simulink model "mrand_bpsk_1u_mp"  (Simulink 6.0)
settings: Solver=ode45  StartTime=0.0  StopTime=" 0.125 - (1/19200)"  RelTol=1e-3
libraries: mspread x4, commutil2 x1, commchan2 x1, commsink2 x1, commseqgen2 x1, commrandsrc2 x1
CloseFcn:
  | clear spreadSigsOut
settings Model: Creator=akansal  LastModifiedBy=mmclerno  ProdHWDeviceType=Specified
settings DataIOCC: SaveTime=off  SignalLoggingName=spreadSigsOut
settings OptimizationCC: BooleanDataType=off  InlineParams=on  MultiInstanced=off
settings FormatCC: IgnoreBidirectionalLines=off
settings HardwareCC: ProdHWDeviceType=Specified
settings CodeAppCC: SimulinkBlockComments=off
settings GRTTargetCC: TargetFcnLib=iso_c_tmw.mat

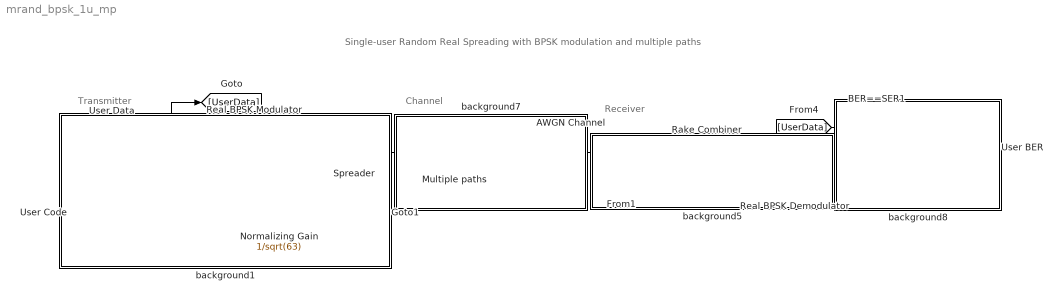
== system mrand_bpsk_1u_mp ==
  note: Single-user Random Real Spreading with BPSK modulation and multiple paths
  note: Transmitter
  note: Channel
  note: Receiver
  " " : commutil2/Unipolar to Bipolar Converter  M=2  polarity=Negative
  AWGN Channel : commchan2/AWGN Channel  seed=1237  noiseMode="Signal to noise ratio  (SNR)"  EbNodB=10  EsNodB=25  SNRdB=5  bitsPerSym=1  Ps=1  Tsym=ts  variance=1
  BER==SER1 : commsink2/Error Rate Calculation  N=0  st_delay=0  cp_mode=Entire frame  subframe=[]  PMode=Port  WsName=ErrorVec  RsMode2=off  stop=off  numErr=100  maxBits=1e6
  Multiple paths : mspread/Multiple paths  p=3  pd=[0 2 6]  ts=1/19200
  Normalizing Gain : Gain  Gain=1/sqrt(63)  SaturateOnIntegerOverflow=on
  Rake Combiner : mspread/Rake Combiner  pd=[0 2 6]  pgain=63
  Real BPSK Demodulator : mspread/Real BPSK Demodulator
  Real BPSK Modulator : mspread/Real BPSK Modulator
  Spreader : Product  SaturateOnIntegerOverflow=on  InputSameDT=on
  User BER : Display
  User Code : Subsystem  BlockChoice=PN Sequence Generator
      link override Gold Sequence Generator: index=7  ts=1/(9600*2*63)  frameBased=on  sampPerFrame=63
      link override Kasami Sequence Generator: codeIdx=4  ts=1/(9600*2*63)  frameBased=on  sampPerFrame=63
      link override PN Sequence Generator: Ts=1/(19200*63)  frameBased=on  sampPerFrame=63
      settings: AttributesFormatString=%<BlockChoice>  TemplateBlock=randcodes/Configurable System  MemberBlocks=Gold Sequence Generator,Kasami Sequence Generator,PN Sequence Generator
  User Data : commrandsrc2/Random Integer Generator  mul=2  seed=37  Ts=1/19200  frameBased=on  sampPerFrame=1  orient=off
  background1 : Subsystem
      mask Display: disp('')
  background5 : Subsystem
      mask Display: disp('')
  background7 : Subsystem  Orientation=up
      mask Display: disp('')
  background8 : Subsystem
      mask Display: disp('')
  wires:
  User Data/1 -> [UserData], Real BPSK Modulator/1
  Real BPSK Modulator/1 -> Spreader/1
  Multiple paths/1 -> AWGN Channel/1
  " "/1 -> Normalizing Gain/1
  Normalizing Gain/1 -> Spreader/2, [UserCode]
  AWGN Channel/1 -> Rake Combiner/1
  Spreader/1 -> Multiple paths/1
  BER==SER1/1 -> User BER/1
  Real BPSK Demodulator/1 -> BER==SER1/2
  Rake Combiner/1 -> Real BPSK Demodulator/1
  [UserCode] -> Rake Combiner/2
  [UserData] -> BER==SER1/1
  User Code/1(Out1) -> " "/1

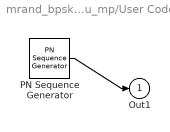
== system mrand_bpsk_1u_mp/User Code ==
  PN Sequence Generator : commseqgen2/PN Sequence Generator  poly=[1 0 0 0 0 1 1]  ini_sta=[0 0 0 0 0 1]  shift=0  Ts=1/(19200*63)  frameBased=on  sampPerFrame=63  reset=off
  Out1 : Outport
  wires:
  PN Sequence Generator/1 -> Out1/1

== system mrand_bpsk_1u_mp/background1 ==

== system mrand_bpsk_1u_mp/background5 ==

== system mrand_bpsk_1u_mp/background7 ==

== system mrand_bpsk_1u_mp/background8 ==
